simulink model "sim_control_pd_2DOF"  (R2019b)
settings: Solver=VariableStepAuto  StartTime=0.0  StopTime=10.0  RelTol=1e-3
values from neighbouring files (symbols this model uses):
  q0 = [90*pi/180;0;0;0]    [control_pd_g.m]
  q_ = [110*pi/180;-30*pi/180;0;0]    [control_pd_g.m]
  theta = load('../theta.mat').theta    [control_pd_g.m]    (also in modelo_dinamico_lineal.m)
undefined symbols (not defined in the file or in its folder): K, u_
settings Model: Creator=AlejnadroZapett  LastModifiedBy=AlejnadroZapett

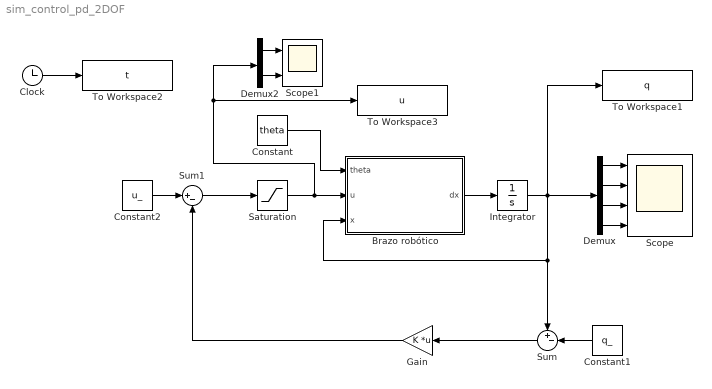
== system sim_control_pd_2DOF ==
  Brazo robótico : MATLAB Function  TreatAsAtomicUnit=on
  Clock : Clock
  Constant : Constant  Value=theta
  Constant1 : Constant  Value=q_
  Constant2 : Constant  Value=u_
  Demux : Demux
  Demux2 : Demux  Outputs=2
  Gain : Gain  Gain=K  Multiplication=Matrix(K*u) (u vector)
  Integrator : Integrator  InitialCondition=q0
  Saturation : Saturate  UpperLimit=255  LowerLimit=-255
  Scope : Scope  NumInputPorts=4
  Scope1 : Scope  NumInputPorts=2
  Sum : Sum  Inputs=+-|
  Sum1 : Sum  Inputs=|+-
  To Workspace1 : ToWorkspace  VariableName=q  SampleTime=-1
  To Workspace2 : ToWorkspace  VariableName=t  SampleTime=-1
  To Workspace3 : ToWorkspace  VariableName=u  SampleTime=-1
  wires:
  Brazo robótico/1(dx) -> Integrator/1
  Integrator/1 -> To Workspace1/1, Demux/1, Brazo robótico/3(x), Sum/1
  Constant/1 -> Brazo robótico/1(theta)
  Constant1/1 -> Sum/2
  Sum/1 -> Gain/1
  Gain/1 -> Sum1/2
  Constant2/1 -> Sum1/1
  Demux/1 -> Scope/1
  Demux/4 -> Scope/4
  Demux/3 -> Scope/3
  Demux/2 -> Scope/2
  Demux2/1 -> Scope1/1
  Demux2/2 -> Scope1/2
  Saturation/1 -> To Workspace3/1, Demux2/1, Brazo robótico/2(u)
  Sum1/1 -> Saturation/1
  Clock/1 -> To Workspace2/1

== matlab function sim_control_pd_2DOF/Brazo robótico ==
  data: theta input; u input; dx output; x input
function dx = fcn(theta,u,x)

dx = zeros(4,1);

u1 = u(1);
u2 = u(2);

q1 = x(1);
q2 = x(2);
dq1 = x(3);
dq2 = x(4);

M11 = (theta(1) + theta(2)*cos(q1));
M12 = (theta(3) + theta(4)*cos(q2));
M21 = (theta(11) + theta(12)*cos(q2));
M22 = theta(13);

C11 = theta(5)*sin(q2)*dq2;
C12 = theta(6)*sin(q2)*dq2;
C21 = theta(14)*sin(q2)*dq1;
C22 = 0;

G1 = theta(7)*cos(q1)+theta(8)*cos(q1+q2);
G2 = theta(14)*cos(q1+q2);

% F1 = theta(9)*dq1 + theta(10)*sign(dq1);
% F2 = theta(16)*dq2 + theta(17)*sign(dq2);
F1 = theta(9)*dq1;
F2 = theta(16)*dq2;

M = [M11 M12;M21 M22];
C = [C11 C12;C21 C22];
G = [G1;G2];
F = [F1;F2];
T = [u1;u2];

D = -inv(M)*(C*[dq1;dq2]+G+F-T);

dx(1) = dq1;
dx(2) = dq2;
dx(3) = D(1);
dx(4) = D(2);
